simulink model "aquabot_view"  (R2023b)
settings: Solver=FixedStepAuto  StartTime=0.0  StopTime=Inf  RelTol=1e-3
model workspace (MAT data in the model file):
  SL_ROS_VariableLengthArrays_MaxSizes.CommonInfo.ArrayTruncateAction = 'EmitWarning'
  SL_ROS_VariableLengthArrays_MaxSizes.MsgTypeMap = containers.Map
  SL_ROS_VariableLengthArrays_MaxSizes.MsgTypeMap.serialization.keys = {'sensor_msgs/Image', 'sensor_msgs/PointCloud2'}
  SL_ROS_VariableLengthArrays_MaxSizes.MsgTypeMap.serialization.values{1}(1).PropertyName = 'data'
  SL_ROS_VariableLengthArrays_MaxSizes.MsgTypeMap.serialization.values{1}(1).DataType = 'uint8'
  SL_ROS_VariableLengthArrays_MaxSizes.MsgTypeMap.serialization.values{1}(1).MaxLength = 1244160
  SL_ROS_VariableLengthArrays_MaxSizes.MsgTypeMap.serialization.values{1}(2).PropertyName = 'encoding'
  SL_ROS_VariableLengthArrays_MaxSizes.MsgTypeMap.serialization.values{1}(2).DataType = 'uint8'
  SL_ROS_VariableLengthArrays_MaxSizes.MsgTypeMap.serialization.values{1}(2).MaxLength = 128
  SL_ROS_VariableLengthArrays_MaxSizes.MsgTypeMap.serialization.values{2}(1).PropertyName = 'data'
  SL_ROS_VariableLengthArrays_MaxSizes.MsgTypeMap.serialization.values{2}(1).DataType = 'uint8'
  SL_ROS_VariableLengthArrays_MaxSizes.MsgTypeMap.serialization.values{2}(1).MaxLength = 960000
  SL_ROS_VariableLengthArrays_MaxSizes.MsgTypeMap.serialization.values{2}(2).PropertyName = 'fields'
  SL_ROS_VariableLengthArrays_MaxSizes.MsgTypeMap.serialization.values{2}(2).DataType = 'sensor_msgs/PointField'
  SL_ROS_VariableLengthArrays_MaxSizes.MsgTypeMap.serialization.values{2}(2).MaxLength = 16
  SL_ROS_VariableLengthArrays_MaxSizes.MsgTypeMap.serialization.uniformity = 0
  SL_ROS_VariableLengthArrays_MaxSizes.MsgTypeMap.serialization.keyType = 'char'
  SL_ROS_VariableLengthArrays_MaxSizes.MsgTypeMap.serialization.valueType = 'any'
undefined symbols (not defined in the file or in its folder): pose
libraries: ros2lib x11
settings Model: Creator=nicolas  LastModifiedBy=nicolas
settings OptimizationCC: EnhancedBackFolding=on  PassReuseOutputArgsAs=Individual arguments  ZeroExternalMemoryAtStartup=off  ZeroInternalMemoryAtStartup=off  InitFltsAndDblsToZero=on  MaxStackSize=64  OptimizeBlockOrder=speed  DifferentSizesBufferReuse=on  OptimizationCustomize=off  EfficientTunableParamExpr=on
settings DebuggingCC: ParameterTunabilityLossMsg=error
settings HardwareCC: ProdBitPerLong=64  ProdLongLongMode=on  ProdHWDeviceType=Intel->x86-64 (Linux 64)  TargetLongLongMode=on  UseEmbeddedCoderFeatures=off
settings SFSimCC: SimTargetLang=C++  SimGPUStackLimitPerThread=4096  SimGPUErrorChecks=on
settings RTWCC: Description=Embedded Coder  SystemTargetFile=ert.tlc  HardwareBoard=Robot Operating System 2 (ROS 2)  TLCOptions="-aInlineSetEventsForThisBaseRateFcn=TLC_FALSE -aSuppressMultiTaskScheduler=TLC_FALSE  -aRateBasedStepFcn=0"  TemplateMakefile=ert_default_tmf  Toolchain=Colcon Tools  BuildConfiguration=Faster Runs  TargetLang=C++
settings CodeAppCC: ForceParamTrailComments=on  IgnoreCustomStorageClasses=off  OperatorAnnotations=on  SimulinkDataObjDesc=on  SFDataObjDesc=on  InsertBlockDesc=on
settings ERTTargetCC: CodeInterfacePackaging=C++ class  SupportNonInlinedSFcns=on  RootIOFormat=Structure reference

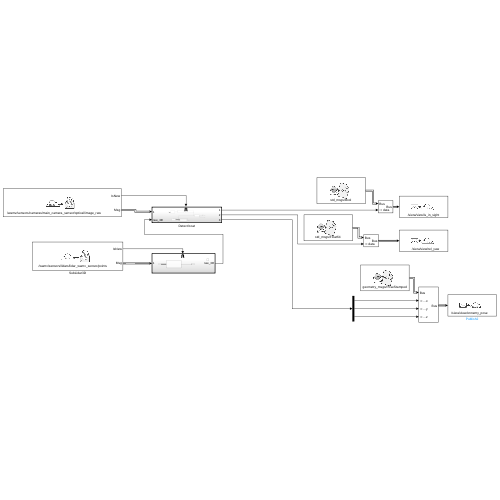
[thumbnail: Simulink's stored preview of the top-level diagram]
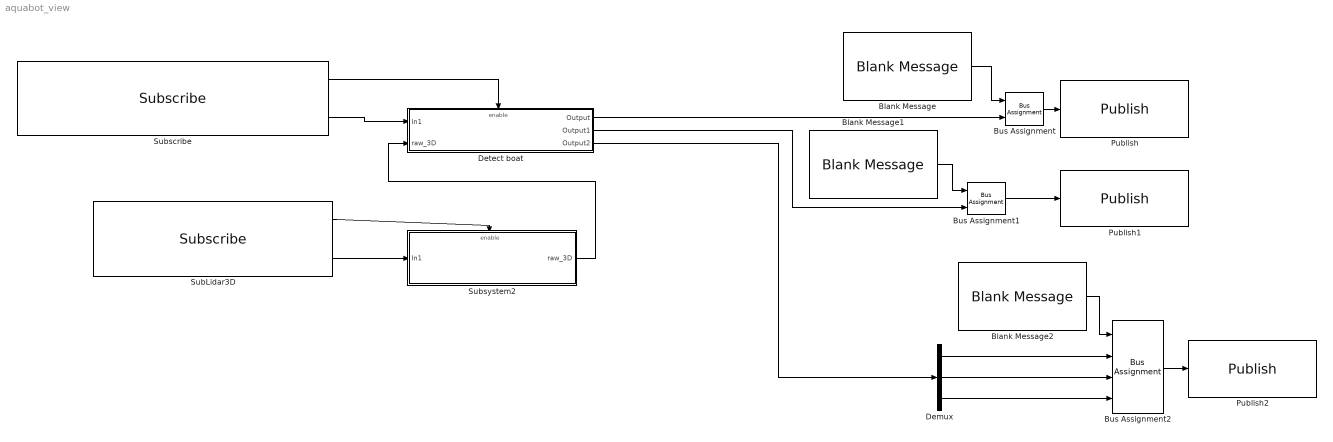
== system aquabot_view ==
  Blank Message : ros2lib/Blank Message  messageClass=Message  entityType=std_msgs/Bool  messageType=std_msgs/Bool  SampleTime=inf
  Blank Message1 : ros2lib/Blank Message  messageClass=Message  entityType=std_msgs/Float64  messageType=std_msgs/Float64  SampleTime=inf
  Blank Message2 : ros2lib/Blank Message  messageClass=Message  entityType=geometry_msgs/PoseStamped  messageType=geometry_msgs/PoseStamped  SampleTime=inf
  Bus Assignment : BusAssignment  AssignedSignals=data
  Bus Assignment1 : BusAssignment  AssignedSignals=data
  Bus Assignment2 : BusAssignment  AssignedSignals=pose.position.x,pose.position.y,pose.position.z
  Demux : Demux  Outputs=3
  Detect boat : Subsystem
  Publish : ros2lib/Publish  topicSource=Specify your own  topic=/siera/view/is_in_sight  messageType=std_msgs/Bool  QOSHistory=Keep last  QOSDepth=1  QOSReliability=Reliable  QOSDurability=Volatile
  Publish1 : ros2lib/Publish  topicSource=Specify your own  topic=/siera/view/rel_yaw  messageType=std_msgs/Float64  QOSHistory=Keep last  QOSDepth=1  QOSReliability=Reliable  QOSDurability=Volatile
  Publish2 : ros2lib/Publish  topicSource=Specify your own  topic=/siera/view/ennemy_pose  messageType=geometry_msgs/PoseStamped  QOSHistory=Keep last  QOSDepth=1  QOSReliability=Reliable  QOSDurability=Volatile
  SubLidar3D : ros2lib/Subscribe  topicSource=Select from ROS network  topic=/wamv/sensors/lidars/lidar_wamv_sensor/points  messageType=sensor_msgs/PointCloud2  sampleTime=-1  QOSHistory=Keep last  QOSDepth=1  QOSReliability=Reliable  QOSDurability=Volatile
  Subscribe : ros2lib/Subscribe  topicSource=Select from ROS network  topic=/wamv/sensors/cameras/main_camera_sensor/optical/image_raw  messageType=sensor_msgs/Image  sampleTime=-1  QOSHistory=Keep last  QOSDepth=1  QOSReliability=Reliable  QOSDurability=Volatile
  Subsystem2 : Subsystem
  wires:
  SubLidar3D/2 -> Subsystem2/1(In1)
  Subscribe/2 -> Detect boat/1(In1)
  Subscribe/1 -> Detect boat/Enable
  SubLidar3D/1 -> Subsystem2/Enable
  Subsystem2/1(raw_3D) -> Detect boat/2(raw_3D)
  Bus Assignment/1 -> Publish/1
  Blank Message/1 -> Bus Assignment/1
  Detect boat/1(Output) -> Bus Assignment/2
  Detect boat/2(Output1) -> Bus Assignment1/2
  Bus Assignment1/1 -> Publish1/1
  Blank Message1/1 -> Bus Assignment1/1
  Demux/2 -> Bus Assignment2/3
  Bus Assignment2/1 -> Publish2/1
  Detect boat/3(Output2) -> Demux/1
  Blank Message2/1 -> Bus Assignment2/1
  Demux/3 -> Bus Assignment2/4
  Demux/1 -> Bus Assignment2/2

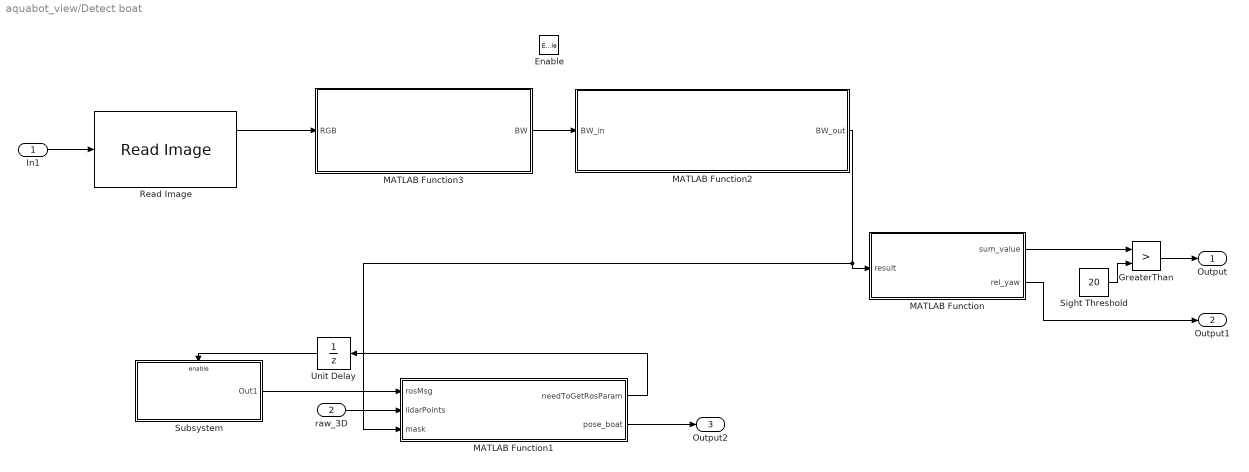
== system aquabot_view/Detect boat ==
  In1 : Inport
  raw_3D : Inport  Port=2
  Enable : EnablePort
  GreaterThan : RelationalOperator  Operator=>  OutDataTypeStr=boolean  RndMeth=Simplest  InputSameDT=off
  MATLAB Function : MATLAB Function  TreatAsAtomicUnit=on
  MATLAB Function1 : MATLAB Function  TreatAsAtomicUnit=on
  MATLAB Function2 : MATLAB Function  TreatAsAtomicUnit=on
  MATLAB Function3 : MATLAB Function  TreatAsAtomicUnit=on
  Read Image : ros2lib/Read Image  MaximumImageSize=[576, 720]  ImageEncoding=rgb8  ShowAlphaOutput=off  ShowErrorCodeOutput=on  VariableSizeOutputs=off
  Sight Threshold : Constant  Value=20
  Subsystem : Subsystem
  Unit Delay : UnitDelay  InitialCondition=1  SampleTime=-1  HasFrameUpgradeWarning=on
  Output : Outport
  Output1 : Outport  Port=2
  Output2 : Outport  Port=3
  wires:
  Read Image/1 -> MATLAB Function3/1(RGB)
  MATLAB Function2/1(BW_out) -> MATLAB Function1/3(mask), MATLAB Function/1(result)
  MATLAB Function3/1(BW) -> MATLAB Function2/1(BW_in)
  In1/1 -> Read Image/1
  MATLAB Function/1(sum_value) -> GreaterThan/1
  Sight Threshold/1 -> GreaterThan/2
  Subsystem/1(Out1) -> MATLAB Function1/1(rosMsg)
  MATLAB Function1/1(needToGetRosParam) -> Unit Delay/1
  Unit Delay/1 -> Subsystem/Enable
  raw_3D/1 -> MATLAB Function1/2(lidarPoints)
  MATLAB Function1/2(pose_boat) -> Output2/1
  GreaterThan/1 -> Output/1
  MATLAB Function/2(rel_yaw) -> Output1/1

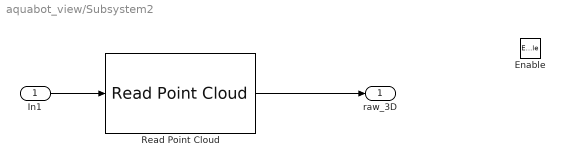
== system aquabot_view/Subsystem2 ==
  In1 : Inport
  Enable : EnablePort
  Read Point Cloud : ros2lib/Read Point Cloud  MaximumPointCloudSize=[16, 1875]  PreserveStructure=off  ShowRGBOutput=off  ShowIntensityOutput=off  ShowErrorCodeOutput=off  VariableSizeOutputs=off
  raw_3D : Outport
  wires:
  Read Point Cloud/1 -> raw_3D/1
  In1/1 -> Read Point Cloud/1

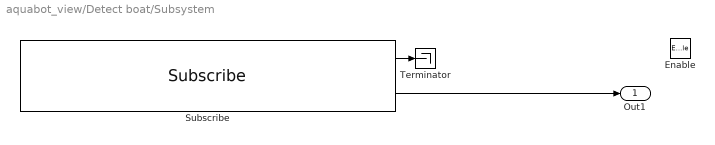
== system aquabot_view/Detect boat/Subsystem ==
  Enable : EnablePort
  Subscribe : ros2lib/Subscribe  topicSource=Select from ROS network  topic=/wamv/sensors/cameras/main_camera_sensor/optical/camera_info  messageType=sensor_msgs/CameraInfo  sampleTime=-1  QOSHistory=Keep last  QOSDepth=1  QOSReliability=Reliable  QOSDurability=Volatile
  Terminator : Terminator
  Out1 : Outport
  wires:
  Subscribe/1 -> Terminator/1
  Subscribe/2 -> Out1/1

== matlab function aquabot_view/Detect boat/MATLAB Function1 ==
  data: rosMsg input; needToGetRosParam output; lidarPoints input; mask input; pose_boat output
function [needToGetRosParam, pose_boat]= projectLidarOnCam(rosMsg, lidarPoints, mask)
    if rosMsg.d_SL_Info.ReceivedLength <= 0
        needToGetRosParam = 1;
        pose_boat = [0 0 0];
        return;
    end
    needToGetRosParam = 0;

    % Filter ground from Lidar
    % pc = pcorganize(pointCloud(lidarPoints), lidarParameters(16, [pi/12 -pi/12], 1875));
    % groundPtsIdx = segmentGroundFromLidarData(pc);
    % nonGroundPtCloud = select(pc,~groundPtsIdx,'OutputSize','full');

    intrinsics = cameraIntrinsicsFromOpenCV(reshape(rosMsg.k,3,3)',rosMsg.d(1:rosMsg.d_SL_Info.ReceivedLength),single([rosMsg.height, rosMsg.width]));
    tform = rigidtform3d([0 -105 90], [0.1 0 -0.2]);
    [imPts, idx] = projectLidarPointsOnImage(lidarPoints,intrinsics,tform);
    
    r_pt = max(round(imPts),1);
    I = sub2ind(size(mask),r_pt(:,2),r_pt(:,1));
    lidar_pt = idx(mask(I)==1,:);

    pose_boat = double(mean(lidarPoints(lidar_pt,:),1));
    pose_boat(isnan(pose_boat)) = 0;
end

== matlab function aquabot_view/Detect boat/MATLAB Function ==
  data: result input; sum_value output; rel_yaw output
function [sum_value, rel_yaw] = checkEnnemy(result)
    sum_value = sum(result, "all");
    
    reg = regionprops(result,'centroid');
    if size(reg, 1) >= 1
        rel_yaw = ((reg(1).Centroid(1)/size(result,2))-0.5) * pi;
    else
        rel_yaw = 0;
    end
end

== matlab function aquabot_view/Detect boat/MATLAB Function2 ==
  data: BW_in input; BW_out output
function BW_out  = filterRegions(BW_in)
%filterRegions Filter BW image using auto-generated code from imageRegionAnalyzer app.

% Auto-generated by imageRegionAnalyzer app on 24-Nov-2023
%---------------------------------------------------------

 BW_out = bwpropfilt(BW_in,'Area',[0 10000]);

 
%  %Load ground truth data from a MAT-file into the workspace. Extract the
% %image and point cloud data from the ground truth data
% dataPath = fullfile(toolboxdir('lidar'),'lidardata','lcc','sampleColoredPtCloud.mat');
% gt  = load(dataPath);
% %img = gt.im;
% img=BW_out;
% pc = gt.ptCloud;
% 
% %Extract the camera intrinsic parameters from the ground truth data
% intrinsics = gt.camParams;
% 
% %Extract the camera to lidar transformation matrix from the ground truth data,
% % and invert to find the lidar to camera transformation matrix
% tform = invert(gt.tform);
% 
% %Downsample the point cloud data
% p1 = pcdownsample(pc,'gridAverage',0.5);
% 
% %Project the point cloud onto the image frame.
% imPts = projectLidarPointsOnImage(p1,intrinsics,tform);
% 
% %Overlay the projected points on the image
% figure
% imshow(img)
% hold on
% plot(imPts(:,1),imPts(:,2),'.','Color','r')
% hold off

== matlab function aquabot_view/Detect boat/MATLAB Function3 ==
  data: RGB input; BW output
function BW = createMask(RGB)
%createMask  Threshold RGB image using auto-generated code from colorThresholder app.
%  [BW,MASKEDRGBIMAGE] = createMask(RGB) thresholds image RGB using
%  auto-generated code from the colorThresholder app. The colorspace and
%  range for each channel of the colorspace were set within the app. The
%  segmentation mask is returned in BW, and a composite of the mask and
%  original RGB images is returned in maskedRGBImage.

% Auto-generated by colorThresholder app on 27-Nov-2023
%------------------------------------------------------


% Convert RGB image to chosen color space
I = RGB;

% Define thresholds for channel 1 based on histogram settings
channel1Min = 14.000;
channel1Max = 223.000;

% Define thresholds for channel 2 based on histogram settings
channel2Min = 7.000;
channel2Max = 19.000;

% Define thresholds for channel 3 based on histogram settings
channel3Min = 0.000;
channel3Max = 39.000;

% Create mask based on chosen histogram thresholds
sliderBW = (I(:,:,1) >= channel1Min ) & (I(:,:,1) <= channel1Max) & ...
    (I(:,:,2) >= channel2Min ) & (I(:,:,2) <= channel2Max) & ...
    (I(:,:,3) >= channel3Min ) & (I(:,:,3) <= channel3Max);
BW = sliderBW;

% Initialize output masked image based on input image.
maskedRGBImage = RGB;

% Set background pixels where BW is false to zero.
maskedRGBImage(repmat(~BW,[1 1 3])) = 0;

end
